simulink model "Gesamtmodell_2015b"  (R2015b)
settings: Solver=ode3  StartTime=0.0  StopTime=inf  FixedStep=dt  RelTol=1e-3
undefined symbols (not defined in the file or in its folder): Com1, dt, K1, K2, K3, Kpsi, Kx, Ky, none, sigbuilder_block, Tpsi, Tx, Ty
libraries: xpcrtudplib x9, xpcobsoletelib x4, simulink x2, xpcseriallib x1, slrtlib x1
(part 1 of 3)
CloseFcn:
  | rtwprivate ssgencode ModelCloseRequest Robotino_Strecke_reall_2009
settings Model: SimulationMode=external  Creator=atlabor  LastModifiedBy=atlabor
settings SolverCC: EnableConcurrentExecution=on
settings DataIOCC: LimitDataPoints=off  SaveFormat=Array  SignalLoggingSaveFormat=ModelDataLogs
settings OptimizationCC: BlockReduction=off  OptimizeBlockIOStorage=off  BufferReuse=off  GlobalBufferReuse=off  ExpressionFolding=off  ExpressionDepthLimit=2147483647  LocalBlockOutputs=off  InitFltsAndDblsToZero=on
settings DebuggingCC: SaveWithParameterizedLinksMsg=none  UnderspecifiedInitializationDetection=Classic  MergeDetectMultiDrivingBlocksExec=none  SolverPrmCheckMsg=warning  FcnCallInpInsideContextMsg=EnableAllAsWarning  StateNameClashWarn=warning
settings HardwareCC: ProdBitPerPointer=32  ProdLargestAtomicFloat=None  ProdWordSize=32  ProdLongLongMode=on  ProdHWDeviceType=Generic->32-bit x86 compatible
settings SFSimCC: SimParseCustomCode=off
settings RTWCC: SystemTargetFile=slrt.tlc  TemplateMakefile=slrt_default_tmf  Description=Simulink Real-Time  RTWCompilerOptimization=on
settings ConfigComp: CovModelRefEnable=Off  CovSFcnEnable=off

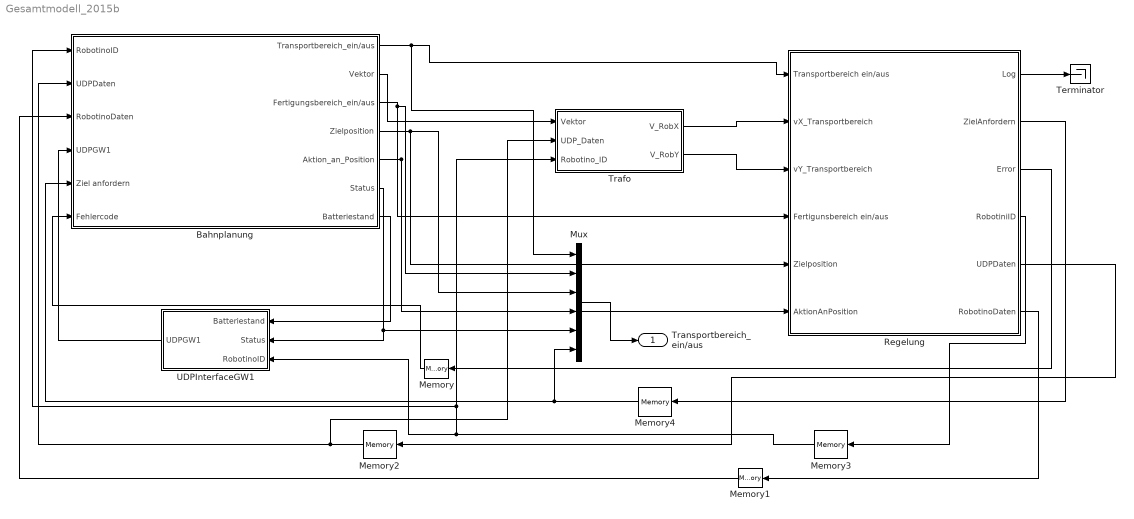
== system Gesamtmodell_2015b ==
  Bahnplanung : Subsystem
  Memory{,1..4} (5 alike) : Memory
  Mux : Mux  Inputs=6
  Regelung : Subsystem
  Terminator : Terminator
  Trafo : MATLAB Function  TreatAsAtomicUnit=on
  UDPInterfaceGW1 : Subsystem
  Transportbereich_ein/aus : Outport
  wires:
  Bahnplanung/1(Transportbereich_ein/aus) -> Mux/1, Regelung/1(Transportbereich ein/aus)
  Bahnplanung/3(Fertigungsbereich_ein/aus) -> Mux/2, Regelung/4(Fertigunsbereich ein/aus)
  Bahnplanung/7(Batteriestand) -> UDPInterfaceGW1/1(Batteriestand)
  Bahnplanung/6(Status) -> UDPInterfaceGW1/2(Status), Mux/5
  UDPInterfaceGW1/1(UDPGW1) -> Bahnplanung/4(UDPGW1)
  Regelung/3(Error) -> Memory/1
  Bahnplanung/4(Zielposition) -> Mux/3, Regelung/5(Zielposition)
  Bahnplanung/5(Aktion_an_Position) -> Mux/4, Regelung/6(AktionAnPosition)
  Regelung/5(UDPDaten) -> Memory2/1
  Regelung/6(RobotinoDaten) -> Memory1/1
  Regelung/1(Log) -> Terminator/1
  Memory/1 -> Bahnplanung/6(Fehlercode)
  Memory1/1 -> Bahnplanung/3(RobotinoDaten)
  Memory3/1 -> UDPInterfaceGW1/3(RobotinoID), Trafo/3(Robotino_ID), Bahnplanung/1(RobotinoID)
  Regelung/2(ZielAnfordern) -> Memory4/1
  Trafo/1(V_RobX) -> Regelung/2(vX_Transportbereich)
  Trafo/2(V_RobY) -> Regelung/3(vY_Transportbereich)
  Bahnplanung/2(Vektor) -> Trafo/1(Vektor)
  Memory2/1 -> Trafo/2(UDP_Daten), Bahnplanung/2(UDPDaten)
  Regelung/4(RobotiniID) -> Memory3/1
  Mux/1 -> Transportbereich_ein/aus/1
  Memory4/1 -> Mux/6, Bahnplanung/5(Ziel anfordern)

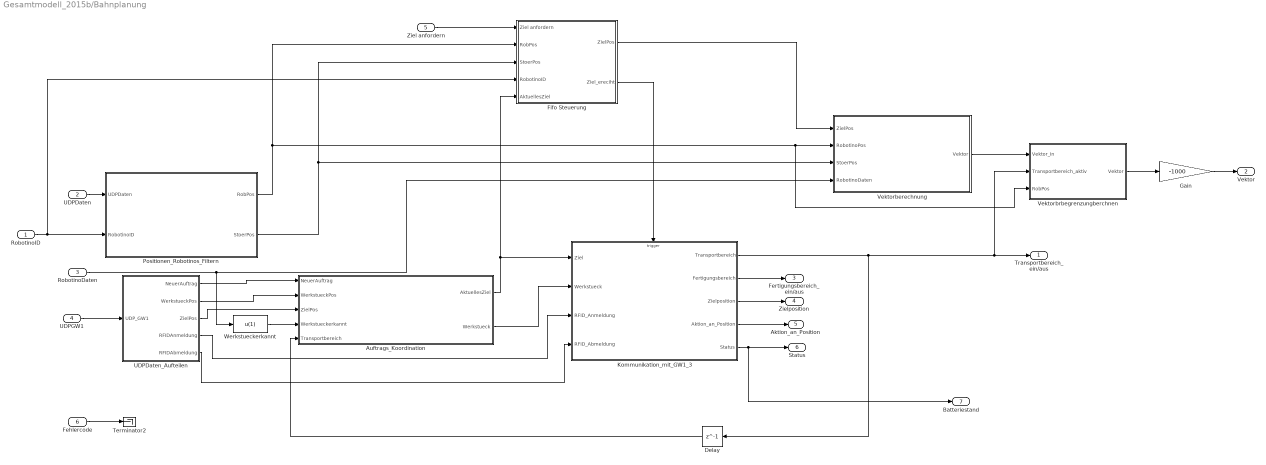
== system Gesamtmodell_2015b/Bahnplanung ==
  RobotinoID : Inport
  UDPDaten : Inport  Port=2  PortDimensions=56
  RobotinoDaten : Inport  Port=3
  UDPGW1 : Inport  Port=4
  Ziel anfordern : Inport  Port=5
  Fehlercode : Inport  Port=6
  Auftrags_Koordination : Stateflow chart  TreatAsAtomicUnit=on
  Delay : Delay  DelayLength=1
  Fifo Steuerung : Subsystem
  Gain : Gain  Gain=-1000
  Kommunikation_mit_GW1_3 : Stateflow chart  TreatAsAtomicUnit=on
  Positionen_Robotinos_Filtern : MATLAB Function  TreatAsAtomicUnit=on
  Terminator2 : Terminator
  UDPDaten_Aufteilen : Subsystem
  Vektorberechnung : Subsystem
  Vektorbrbegrenzungberchnen : MATLAB Function  TreatAsAtomicUnit=on
  Werkstueckerkannt : Fcn  Expr=u(1)
  Transportbereich_ein/aus : Outport
  Vektor : Outport  Port=2  OutDataTypeStr=double  PortDimensions=[1 2]
  Fertigungsbereich_ein/aus : Outport  Port=3
  Zielposition : Outport  Port=4
  Aktion_an_Position : Outport  Port=5
  Status : Outport  Port=6
  Batteriestand : Outport  Port=7
  wires:
  RobotinoID/1 -> Positionen_Robotinos_Filtern/2(RobotinoID), Fifo Steuerung/4(RobotinoID)
  UDPDaten/1 -> Positionen_Robotinos_Filtern/1(UDPDaten)
  Positionen_Robotinos_Filtern/2(StoerPos) -> Fifo Steuerung/3(StoerPos), Vektorberechnung/3(StoerPos)
  RobotinoDaten/1 -> Vektorberechnung/4(RobotinoDaten), Werkstueckerkannt/1
  Kommunikation_mit_GW1_3/3(Zielposition) -> Zielposition/1
  Kommunikation_mit_GW1_3/4(Aktion_an_Position) -> Aktion_an_Position/1
  Kommunikation_mit_GW1_3/2(Fertigungsbereich) -> Fertigungsbereich_ein/aus/1
  Kommunikation_mit_GW1_3/1(Transportbereich) -> Delay/1, Transportbereich_ein/aus/1, Vektorbrbegrenzungberchnen/2(Transportbereich_aktiv)
  UDPGW1/1 -> UDPDaten_Aufteilen/1(UDP_GW1)
  UDPDaten_Aufteilen/4(RFIDAnmeldung) -> Kommunikation_mit_GW1_3/3(RFID_Anmeldung)
  UDPDaten_Aufteilen/5(RFIDAbmeldung) -> Kommunikation_mit_GW1_3/4(RFID_Abmeldung)
  UDPDaten_Aufteilen/2(WerkstueckPos) -> Auftrags_Koordination/2(WerkstueckPos)
  UDPDaten_Aufteilen/3(ZielPos) -> Auftrags_Koordination/3(ZielPos)
  Auftrags_Koordination/1(AktuellesZiel) -> Fifo Steuerung/5(AktuellesZiel), Kommunikation_mit_GW1_3/1(Ziel)
  Fehlercode/1 -> Terminator2/1
  UDPDaten_Aufteilen/1(NeuerAuftrag) -> Auftrags_Koordination/1(NeuerAuftrag)
  Auftrags_Koordination/2(Werkstueck) -> Kommunikation_mit_GW1_3/2(Werkstueck)
  Werkstueckerkannt/1 -> Auftrags_Koordination/4(Werkstueckerkannt)
  Vektorbrbegrenzungberchnen/1(Vektor) -> Gain/1
  Gain/1 -> Vektor/1
  Positionen_Robotinos_Filtern/1(RobPos) -> Vektorbrbegrenzungberchnen/3(RobPos), Vektorberechnung/2(RobotinoPos), Fifo Steuerung/2(RobPos)
  Vektorberechnung/1(Vektor) -> Vektorbrbegrenzungberchnen/1(Vektor_In)
  Ziel anfordern/1 -> Fifo Steuerung/1(Ziel anfordern)
  Fifo Steuerung/1(ZielPos) -> Vektorberechnung/1(ZielPos)
  Fifo Steuerung/2(Ziel_ereciht) -> Kommunikation_mit_GW1_3/Trigger
  Delay/1 -> Auftrags_Koordination/5(Transportbereich)
  Kommunikation_mit_GW1_3/5(Status) -> Batteriestand/1, Status/1

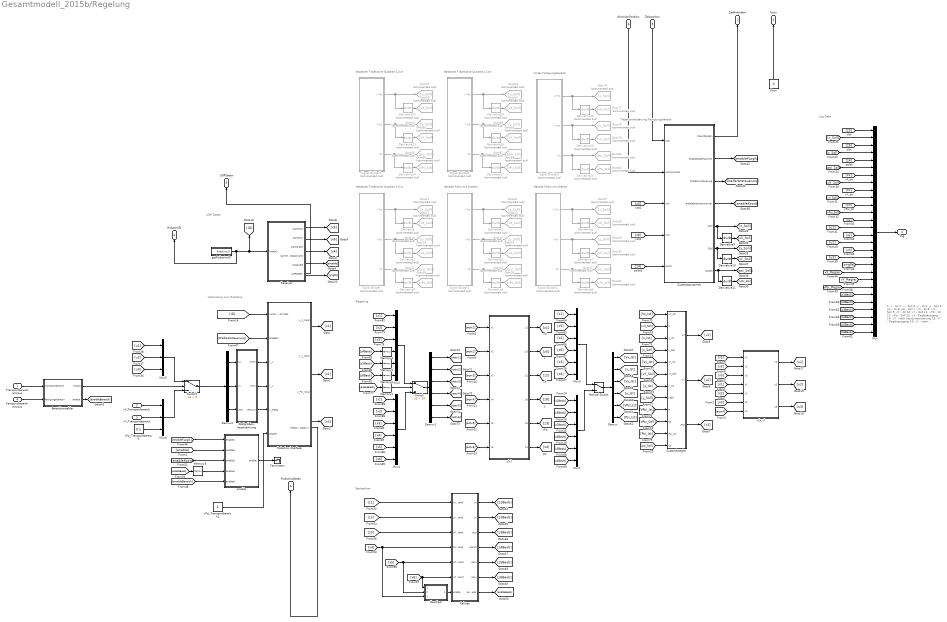
== system Gesamtmodell_2015b/Regelung ==
  note: Trajektorienplanung Fertigungsbereich
  note: Regelung
  note: Verbindung zum Robotino
  note: UDP Daten
  note: Geplante Trajektorie Quadrat 1x1m
  note: Log Data
  note: 1:    x     - Ist
      | 2:    x     - Soll
      | 3:    y     - Ist
      | 4:    y     - Soll
      | 5:   psi   - Ist
      | 6:   psi   - Soll
      | 7:   vX   - Ist
      | 8:   vX   - Soll
      | 9:   vY   - Ist
      | 10: vY   - Soll
      | 11: vPsi - Ist
      | 12: vPsi - Soll
      | 13: vX   - Reglerausgang
      | 14: vX   - nach InputLinearisierung
      | 15: vY   - Reglerausgang
      | 16: vY  - nach InputLinearisierung
      | 17: vPsi - Reglerausgang
      | 18: vPsi - nach InputLinearisierung
      | 19: Kamera Psi
      | 20: vX   - Regler (Geschwindigkeit)
      | 21: vY   - Regler (Geschwindigkeit)
      | 22: vPsi - Regler (Geschwindigkeit)
  note: Gerade Fahrt mit Drehen
  note: Gerade Fahrt mit Drehen
  note: Beobachter
  note: Geplante Trajektorie Quadrat 1x1m
  note: Geplante Trajektorie Quadrat 1x1m
  note: hinter Fertigungsbereich
  Transportbereich ein/aus : Inport
  vX_Transportbereich : Inport  Port=2
  vY_Transportbereich : Inport  Port=3
  Fertigunsbereich ein/aus : Inport  Port=4
  Zielposition : Inport  Port=5
  AktionAnPosition : Inport  Port=6
  Bereichswaehler : MATLAB Function  TreatAsAtomicUnit=on
  Demux : Demux  Outputs=6
  Demux1 : Demux  Outputs=6
  Demux2 : Demux  Outputs=3
  Derivative{,1..8,12..20} (18 alike) : Derivative  Commented=on
  Derivative10 : Derivative
  Derivative11 : Derivative
  Derivative9 : Derivative
  "Error " : Constant  Value=0
  Goto{11,21,27,52,63,76} (6 alike) : Goto  Commented=on  GotoTag=x_Soll
  Goto{12,22,28,53,64,77} (6 alike) : Goto  Commented=on  GotoTag=vX_Soll
  Goto{13,23,29,54,65,78} (6 alike) : Goto  Commented=on  GotoTag=y_Soll
  Goto{14,24,30,55,66,79} (6 alike) : Goto  Commented=on  GotoTag=vY_Soll
  Goto{15,25,31,56,67,80} (6 alike) : Goto  Commented=on  GotoTag=psi_Soll
  Goto{16,26,32,68..69,81} (6 alike) : Goto  Commented=on  GotoTag=vPsi_Soll
  Kalman : MATLAB Function  TreatAsAtomicUnit=on
  Manual Switch : ManualSwitch
  Memory{1..5} (5 alike) : Memory
  Mux : Mux  Inputs=28
  Mux{1..4} (4 alike) : Mux  Inputs=6
  Mux5 : Mux  Inputs=3
  Mux6 : Mux  Inputs=3
  NewCam : MATLAB Function  TreatAsAtomicUnit=on
  Receiver : Subsystem
  Robotino interface : Subsystem
  Signal Builder : Subsystem  Tag=STV Subsys  Commented=on  LoadFcn=sigbuilder_block('load');  StartFcn=sigbuilder_block('start');  StopFcn=sigbuilder_block('stop');  ClipboardFcn=sigbuilder_block('clipboard');  mask(Sigbuilder block){}
      mask help: Simulink:masks:SigbuilderBlock_MD
      mask init:
      | if ~strcmp(get_param(bdroot(gcbh),'SimulationStatus'),'stopped') tuvar = sigbuilder_block('maskInit'); end
      settings: CopyFcn=sigbuilder_block('copy');  DeleteFcn=sigbuilder_block('delete');  ModelCloseFcn=sigbuilder_block('modelClose');  PreSaveFcn=sigbuilder_block('preSave');  PauseFcn=sigbuilder_block('pause');  ContinueFcn=sigbuilder_block('continue');  NameChangeFcn=sigbuilder_block('namechange');  OpenFcn=sigbuilder_block('open',[6 30 1248 660 ]);  CloseFcn=sigbuilder_block('close');
      mask Display: plot(0, 0, 100, 100,[2, 2, 32, 32, 2], [68, 8, 8, 68, 68],[32, 2], [38, 38], [32, 19, 2],[53, 60, 44], [32, 17, 17, 2],[16, 16, 31, 31]);txt = getActiveGroup(gcbh);text(2, 100, txt,'verticalAlignment', 'top');
  Signal Builder1 : Subsystem  Tag=STV Subsys  Commented=on  LoadFcn=sigbuilder_block('load');  StartFcn=sigbuilder_block('start');  StopFcn=sigbuilder_block('stop');  ClipboardFcn=sigbuilder_block('clipboard');  mask(Sigbuilder block){}
      mask help: Simulink:masks:SigbuilderBlock_MD
      mask init:
      | if ~strcmp(get_param(bdroot(gcbh),'SimulationStatus'),'stopped') tuvar = sigbuilder_block('maskInit'); end
      settings: CopyFcn=sigbuilder_block('copy');  DeleteFcn=sigbuilder_block('delete');  ModelCloseFcn=sigbuilder_block('modelClose');  PreSaveFcn=sigbuilder_block('preSave');  PauseFcn=sigbuilder_block('pause');  ContinueFcn=sigbuilder_block('continue');  NameChangeFcn=sigbuilder_block('namechange');  OpenFcn=sigbuilder_block('open',[6 30 1248 660 ]);  CloseFcn=sigbuilder_block('close');
      mask Display: plot(0, 0, 100, 100,[2, 2, 32, 32, 2], [68, 8, 8, 68, 68],[32, 2], [38, 38], [32, 19, 2],[53, 60, 44], [32, 17, 17, 2],[16, 16, 31, 31]);txt = getActiveGroup(gcbh);text(2, 100, txt,'verticalAlignment', 'top');
  Signal Builder2 : Subsystem  Tag=STV Subsys  Commented=on  LoadFcn=sigbuilder_block('load');  StartFcn=sigbuilder_block('start');  StopFcn=sigbuilder_block('stop');  ClipboardFcn=sigbuilder_block('clipboard');  mask(Sigbuilder block){}
      mask help: Simulink:masks:SigbuilderBlock_MD
      mask init:
      | if ~strcmp(get_param(bdroot(gcbh),'SimulationStatus'),'stopped') tuvar = sigbuilder_block('maskInit'); end
      settings: CopyFcn=sigbuilder_block('copy');  DeleteFcn=sigbuilder_block('delete');  ModelCloseFcn=sigbuilder_block('modelClose');  PreSaveFcn=sigbuilder_block('preSave');  PauseFcn=sigbuilder_block('pause');  ContinueFcn=sigbuilder_block('continue');  NameChangeFcn=sigbuilder_block('namechange');  OpenFcn=sigbuilder_block('open',[6 30 1248 660 ]);  CloseFcn=sigbuilder_block('close');
      mask Display: plot(0, 0, 100, 100,[2, 2, 32, 32, 2], [68, 8, 8, 68, 68],[32, 2], [38, 38], [32, 19, 2],[53, 60, 44], [32, 17, 17, 2],[16, 16, 31, 31]);txt = getActiveGroup(gcbh);text(2, 100, txt,'verticalAlignment', 'top');
  Signal Builder3 : Subsystem  Tag=STV Subsys  Commented=on  LoadFcn=sigbuilder_block('load');  StartFcn=sigbuilder_block('start');  StopFcn=sigbuilder_block('stop');  ClipboardFcn=sigbuilder_block('clipboard');  mask(Sigbuilder block){}
      mask help: Simulink:masks:SigbuilderBlock_MD
      mask init:
      | if ~strcmp(get_param(bdroot(gcbh),'SimulationStatus'),'stopped') tuvar = sigbuilder_block('maskInit'); end
      settings: CopyFcn=sigbuilder_block('copy');  DeleteFcn=sigbuilder_block('delete');  ModelCloseFcn=sigbuilder_block('modelClose');  PreSaveFcn=sigbuilder_block('preSave');  PauseFcn=sigbuilder_block('pause');  ContinueFcn=sigbuilder_block('continue');  NameChangeFcn=sigbuilder_block('namechange');  OpenFcn=sigbuilder_block('open',[6 30 1248 660 ]);  CloseFcn=sigbuilder_block('close');
      mask Display: plot(0, 0, 100, 100,[2, 2, 32, 32, 2], [68, 8, 8, 68, 68],[32, 2], [38, 38], [32, 19, 2],[53, 60, 44], [32, 17, 17, 2],[16, 16, 31, 31]);txt = getActiveGroup(gcbh);text(2, 100, txt,'verticalAlignment', 'top');
  Signal Builder4 : Subsystem  Tag=STV Subsys  Commented=on  LoadFcn=sigbuilder_block('load');  StartFcn=sigbuilder_block('start');  StopFcn=sigbuilder_block('stop');  ClipboardFcn=sigbuilder_block('clipboard');  mask(Sigbuilder block){}
      mask help: Simulink:masks:SigbuilderBlock_MD
      mask init:
      | if ~strcmp(get_param(bdroot(gcbh),'SimulationStatus'),'stopped') tuvar = sigbuilder_block('maskInit'); end
      settings: CopyFcn=sigbuilder_block('copy');  DeleteFcn=sigbuilder_block('delete');  ModelCloseFcn=sigbuilder_block('modelClose');  PreSaveFcn=sigbuilder_block('preSave');  PauseFcn=sigbuilder_block('pause');  ContinueFcn=sigbuilder_block('continue');  NameChangeFcn=sigbuilder_block('namechange');  OpenFcn=sigbuilder_block('open',[6 30 1248 660 ]);  CloseFcn=sigbuilder_block('close');
      mask Display: plot(0, 0, 100, 100,[2, 2, 32, 32, 2], [68, 8, 8, 68, 68],[32, 2], [38, 38], [32, 19, 2],[53, 60, 44], [32, 17, 17, 2],[16, 16, 31, 31]);txt = getActiveGroup(gcbh);text(2, 100, txt,'verticalAlignment', 'top');
  Signal Builder5 : Subsystem  Tag=STV Subsys  Commented=on  LoadFcn=sigbuilder_block('load');  StartFcn=sigbuilder_block('start');  StopFcn=sigbuilder_block('stop');  ClipboardFcn=sigbuilder_block('clipboard');  mask(Sigbuilder block){}
      mask help: Simulink:masks:SigbuilderBlock_MD
      mask init:
      | if ~strcmp(get_param(bdroot(gcbh),'SimulationStatus'),'stopped') tuvar = sigbuilder_block('maskInit'); end
      settings: CopyFcn=sigbuilder_block('copy');  DeleteFcn=sigbuilder_block('delete');  ModelCloseFcn=sigbuilder_block('modelClose');  PreSaveFcn=sigbuilder_block('preSave');  PauseFcn=sigbuilder_block('pause');  ContinueFcn=sigbuilder_block('continue');  NameChangeFcn=sigbuilder_block('namechange');  OpenFcn=sigbuilder_block('open',[6 30 1248 660 ]);  CloseFcn=sigbuilder_block('close');
      mask Display: plot(0, 0, 100, 100,[2, 2, 32, 32, 2], [68, 8, 8, 68, 68],[32, 2], [38, 38], [32, 19, 2],[53, 60, 44], [32, 17, 17, 2],[16, 16, 31, 31]);txt = getActiveGroup(gcbh);text(2, 100, txt,'verticalAlignment', 'top');
  "Stellgrößen- beschränkung " : Subsystem
  Switch : Switch  Criteria=u2 > Threshold  Threshold=10
  Switch1 : Switch  Criteria=u2 > Threshold
  Terminator : Terminator
  Zustandsautomat : Subsystem
  Zustandsregler : Subsystem
  "enable " : MATLAB Function  TreatAsAtomicUnit=on
  getRobotinoID : Subsystem
  "u(x,v) " : MATLAB Function  TreatAsAtomicUnit=on
  vPsi_Transportbereich : Constant  Value=0.1
  vPsi_Transportbereich1 : Constant
  z(x) : MATLAB Function  TreatAsAtomicUnit=on
  Log : Outport
  ZielAnfordern : Outport  Port=2
  Error : Outport  Port=3
  RobotiniID : Outport  Port=4
  UDPDaten : Outport  Port=5
  RobotinoDaten : Outport  Port=6
  wires:
  Fertigunsbereich ein/aus/1 -> Bereichswaehler/2(fertigungsbereich)
  Bereichswaehler/2(enable) -> [enableBereich]
  "Error "/1 -> Error/1
  Mux5/1 -> Switch1/1
  [u1] -> Mux5/1
  [GreiferAnsteuerung] -> Robotino interface/2(Grabber)
  Mux/1 -> Log/1
  [enableBereich] -> "enable "/5(enable5)
  Derivative4/1 -> Goto16/1
  Signal Builder/1(X Pos) -> Derivative/1, Goto11/1
  [u2] -> Mux5/2
  [u3] -> Mux5/3
  vPsi_Transportbereich/1 -> Mux6/3
  Zustandsautomat/1(ZielAnfordern) -> ZielAnfordern/1
  Transportbereich ein/aus/1 -> Bereichswaehler/1(transportbereich)
  Mux6/1 -> Switch1/3
  Bereichswaehler/1(modus) -> Switch1/2
  [x3] -> Mux2/3
  [x1] -> "u(x,v) "/4(x1)
  [x3] -> "u(x,v) "/6(x3)
  [z1] -> Mux/7
  [u2] -> Mux/16
  Receiver/5("origAngle ") -> [origPsi]
  Demux2/2 -> "Stellgrößen- beschränkung "/2(vY)
  Demux2/3 -> "Stellgrößen- beschränkung "/3(vPsi)
  Mux1/1 -> Manual Switch/2
  Mux3/1 -> Manual Switch/1
  [v3] -> "u(x,v) "/3(v3)
  Signal Builder5/3(Psi) -> Goto80/1, Derivative20/1
  [z3] -> Kalman/3(vPsiZustand)
  [u3] -> Mux/18
  [z4] -> Mux3/6
  [z1Beob] -> Mux1/1
  [z5Beob] -> Mux1/2
  [z6Beob] -> Mux1/4
  [u1] -> Mux/14
  Signal Builder1/1(X Pos) -> Derivative1/1, Goto21/1
  [origPsi] -> Mux/19
  [z5] -> Mux/1
  "Stellgrößen- beschränkung "/1(vXlim) -> Robotino interface/3(v_x)
  Derivative11/1 -> [vPsi_Soll]
  Derivative10/1 -> [vY_Soll]
  Signal Builder2/3(Psi) -> Derivative8/1, Goto31/1
  Derivative7/1 -> Goto30/1
  Signal Builder3/3(Psi) -> Goto56/1, Derivative14/1
  Signal Builder1/2(Y Pos) -> Derivative2/1, Goto23/1
  [z6] -> Zustandsautomat/4(yIst)
  Zustandsautomat/2(enableStateMachine) -> [enableFLogik]
  [v3] -> Mux/17
  Receiver/4(CameraSignalValid) -> [enable]
  [psi_Soll] -> Zustandsregler/12("psi_Soll ")
  [z6] -> Mux/3
  Receiver/3("CameraPsi ") -> [x4]
  [vPsi_Soll] -> Mux/12
  z(x)/6(z4) -> [z4]
  vX_Transportbereich/1 -> Mux6/1
  [z2Beob] -> Mux/24
  [z6Beob] -> Mux/28
  [z2] -> Mux3/3
  [z5] -> Mux3/2
  [z4Beob] -> Mux1/6
  [vY_Soll] -> Mux/10
  [vX_Soll] -> Mux/8
  Signal Builder4/3(Psi) -> Goto67/1, Derivative17/1
  Derivative9/1 -> [vX_Soll]
  Memory5/1 -> "enable "/4(enable4)
  Robotino interface/3("v_Psi_lokal ") -> [x3]
  [x2] -> "u(x,v) "/5(x2)
  Robotino interface/2("v_Y_lokal ") -> [x2]
  z(x)/2(z5) -> [z5]
  [z3] -> Mux/11
  [z2] -> Mux/9
  [x5] -> Kalman/5(xZustand), NewCam/2(xZustand)
  Zustandsregler/1(vX) -> [v1]
  Zustandsregler/2(vY) -> [v2]
  Kalman/2(vy) -> [z2Beob]
  [z3Beob] -> Mux/25
  [Psi_Ist] -> Zustandsregler/11(Psi_ist)
  [z1] -> Kalman/1(vxZustand)
  [VPsi_Ist] -> Zustandsregler/9(vPsi_ist)
  Zustandsautomat/3(GreiferAnsteuerung) -> [GreiferAnsteuerung]
  vY_Transportbereich/1 -> Mux6/2
  [x2] -> Mux2/2
  Mux4/1 -> Switch/3
  Demux1/2 -> [actx2]
  Demux1/1 -> [actx1]
  Kalman/4(pospsi) -> [z4Beob]
  [z3Beob] -> Mux1/5
  NewCam/1(enable) -> Kalman/7(enable)
  [ID] -> Robotino interface/1(number of robot)
  Zustandsregler/3("vPsi ") -> [v3]
  Manual Switch/1 -> Demux/1
  Memory4/1 -> Mux2/4
  [enableBeob] -> Memory1/1
  [x6] -> NewCam/1(yZustand), Kalman/6(yZustand)
  Signal Builder3/2(Y Pos) -> Goto54/1, Derivative13/1
  [vY_Soll] -> Zustandsregler/6("vY_Soll ")
  Derivative/1 -> Goto12/1
  [x_Soll] -> Zustandsregler/4(x_Soll)
  Demux1/3 -> [actx3]
  [vY_Regler] -> Mux/21
  Zustandsautomat/6(YSoll) -> [y_Soll], Derivative10/1
  [vX_Soll] -> Zustandsregler/2("vX_Soll ")
  "Stellgrößen- beschränkung "/3(vPsiLim) -> Robotino interface/5(v_theta)
  z(x)/4(z6) -> [z6]
  z(x)/5(z3) -> [z3]
  Zustandsautomat/7(psiSoll) -> [psi_Soll], Derivative11/1
  [enableFLogik] -> "enable "/1(enable1)
  [z5] -> Zustandsautomat/3(xIst)
  AktionAnPosition/1 -> Zustandsautomat/2(AktionAnZiel)
  [z4Beob] -> Mux/26
  [z5Beob] -> Mux/27
  [z2] -> Kalman/2(vyZustand)
  Signal Builder4/1(X Pos) -> Goto63/1, Derivative15/1
  Zustandsautomat/5(xSoll) -> Derivative9/1, [x_Soll]
  Mux2/1 -> Switch/1
  Switch/1 -> Demux1/1
  [actx2] -> z(x)/2(x2)
  [actx3] -> z(x)/3(x3)
  [actx5] -> z(x)/5(x5)
  [actx1] -> z(x)/1(x1)
  Zielposition/1 -> Zustandsautomat/1("Ziel ")
  [z4] -> Zustandsautomat/5(psiIst)
  [z3] -> Mux3/5
  Demux/1 -> [Vx_Ist]
  Signal Builder4/2(Y Pos) -> Goto65/1, Derivative16/1
  [actx6] -> z(x)/6(x6)
  Receiver/1(CameraX) -> [x5]
  Receiver/2(CameraY) -> [x6]
  [vPsi_Soll] -> Zustandsregler/10(vPsi_Soll)
  [x_Soll] -> Mux/2
  [x4] -> Mux4/4
  [x5] -> Mux4/5
  Signal Builder3/1(X Pos) -> Goto52/1, Derivative12/1
  [y_Soll] -> Zustandsregler/8(ySoll)
  Demux1/5 -> [actx5]
  Demux1/4 -> [actx4]
  [z6Beob] -> Memory2/1
  Demux1/6 -> [actx6]
  Zustandsautomat/4(enableStationsnummer) -> [enableKoord]
  [enableKoord] -> "enable "/3(enable3)
  Robotino interface/1(v_X_lokal) -> [x1]
  "Stellgrößen- beschränkung "/2(vYlim) -> Robotino interface/4(v_y)
  z(x)/1(z1) -> [z1]
  Derivative18/1 -> Goto77/1
  Derivative19/1 -> Goto79/1
  Derivative20/1 -> Goto81/1
  Memory3/1 -> Mux2/5
  [z4Beob] -> Memory4/1
  [enableBeob] -> Memory5/1
  Derivative12/1 -> Goto53/1
  Derivative14/1 -> Goto69/1
  Derivative8/1 -> Goto32/1
  [vPsi_Regler] -> Mux/22
  Demux/2 -> [x_Ist]
  [Vx_Ist] -> Zustandsregler/1(vX_Ist)
  Signal Builder/2(Y Pos) -> Derivative3/1, Goto13/1
  Kalman/6(posy) -> [z6Beob]
  Kalman/1(vx) -> [z1Beob]
  Kalman/5(posx) -> [z5Beob]
  Memory1/1 -> Switch/2
  Signal Builder5/1(X Pos) -> Goto76/1, Derivative18/1
  [psi_Soll] -> Mux/6
  z(x)/3(z2) -> [z2]
  [v2] -> "u(x,v) "/2(v2)
  [v1] -> "u(x,v) "/1(v1)
  [z1] -> Mux3/1
  [z6] -> Mux3/4
  "u(x,v) "/2(u2) -> [u2]
  "u(x,v) "/3(u3) -> [u3]
  "u(x,v) "/1(u1) -> [u1]
  [v1] -> Mux/13
  [v2] -> Mux/15
  Derivative15/1 -> Goto64/1
  Derivative17/1 -> Goto68/1
  Derivative16/1 -> Goto66/1
  Derivative13/1 -> Goto55/1
  [z2Beob] -> Mux1/3
  [z1Beob] -> Mux/23
  Kalman/3(vpsi) -> [z3Beob]
  Derivative2/1 -> Goto24/1
  Signal Builder/3(Psi) -> Derivative4/1, Goto15/1
  Derivative3/1 -> Goto14/1
  getRobotinoID/1(Robotino.ID) -> [ID], Receiver/1("RoboID "), RobotiniID/1
  [actx4] -> z(x)/4(x4)
  Kalman/7(enableBeob) -> [enableBeob]
  [x1] -> Mux4/1
  [x3] -> Mux4/3
  [x2] -> Mux4/2
  Derivative6/1 -> Goto28/1
  Signal Builder2/2(Y Pos) -> Derivative7/1, Goto29/1
  Signal Builder5/2(Y Pos) -> Goto78/1, Derivative19/1
  [x6] -> Mux4/6
  [x1] -> Mux2/1
  [x4] -> Kalman/4(PsiZustand), NewCam/3(psiZustand)
  Derivative5/1 -> Goto26/1
  Demux2/1 -> "Stellgrößen- beschränkung "/1(vX)
  [actx4] -> "u(x,v) "/7(x4)
  Demux/4 -> [y_Ist]
  Demux/3 -> [Vy_Ist]
  Memory2/1 -> Mux2/6
  [z5Beob] -> Memory3/1
  Signal Builder2/1(X Pos) -> Derivative6/1, Goto27/1
  Signal Builder1/3(Psi) -> Derivative5/1, Goto25/1
  Demux/5 -> [VPsi_Ist]
  Demux/6 -> [Psi_Ist]
  [x_Ist] -> Zustandsregler/3(x_Ist)
  Derivative1/1 -> Goto22/1
  [y_Soll] -> Mux/4
  [z4] -> Mux/5
  [enable] -> "enable "/2(enable2)
  [vX_Regler] -> Mux/20
  [Vy_Ist] -> Zustandsregler/5(vY_Ist)
  [y_Ist] -> Zustandsregler/7(y_Ist)
  Receiver/6(UDPDaten) -> UDPDaten/1
  Robotino interface/4(RobotinoDaten 1) -> RobotinoDaten/1
  vPsi_Transportbereich1/1 -> Robotino interface/6(enable)
  "enable "/1(enable) -> Terminator/1
  Switch1/1 -> Demux2/1

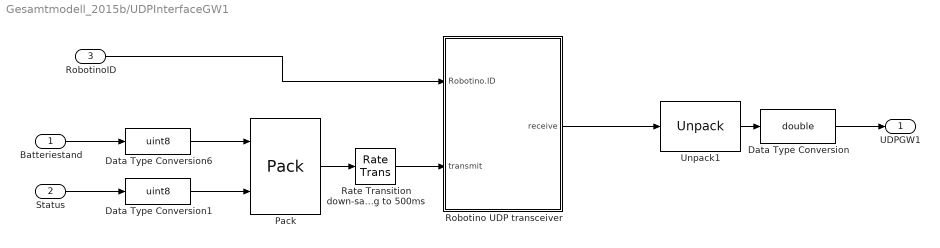
== system Gesamtmodell_2015b/UDPInterfaceGW1 ==
  Batteriestand : Inport
  Status : Inport  Port=2
  RobotinoID : Inport  Port=3
  Data Type Conversion : DataTypeConversion  OutDataTypeStr=double
  Data Type Conversion1 : DataTypeConversion  OutDataTypeStr=uint8
  Data Type Conversion6 : DataTypeConversion  OutDataTypeStr=uint8
  Pack : xpcobsoletelib/Utilities/Pack   datatypes={'uint8','uint8'}  byteAlign=1
  Rate Transition down-sampling to 500ms : RateTransition  OutPortSampleTime=0.5
  Robotino UDP transceiver : Subsystem
  Unpack1 : xpcobsoletelib/Utilities/Unpack   dimensions={[8]}  datatypes={'int8'}  byteAlign=1
  UDPGW1 : Outport
  wires:
  Pack/1 -> Rate Transition down-sampling to 500ms/1
  Data Type Conversion1/1 -> Pack/2
  Data Type Conversion6/1 -> Pack/1
  Batteriestand/1 -> Data Type Conversion6/1
  Status/1 -> Data Type Conversion1/1
  Robotino UDP transceiver/1(receive) -> Unpack1/1
  Rate Transition down-sampling to 500ms/1 -> Robotino UDP transceiver/2(transmit)
  RobotinoID/1 -> Robotino UDP transceiver/1(Robotino.ID)
  Unpack1/1 -> Data Type Conversion/1
  Data Type Conversion/1 -> UDPGW1/1

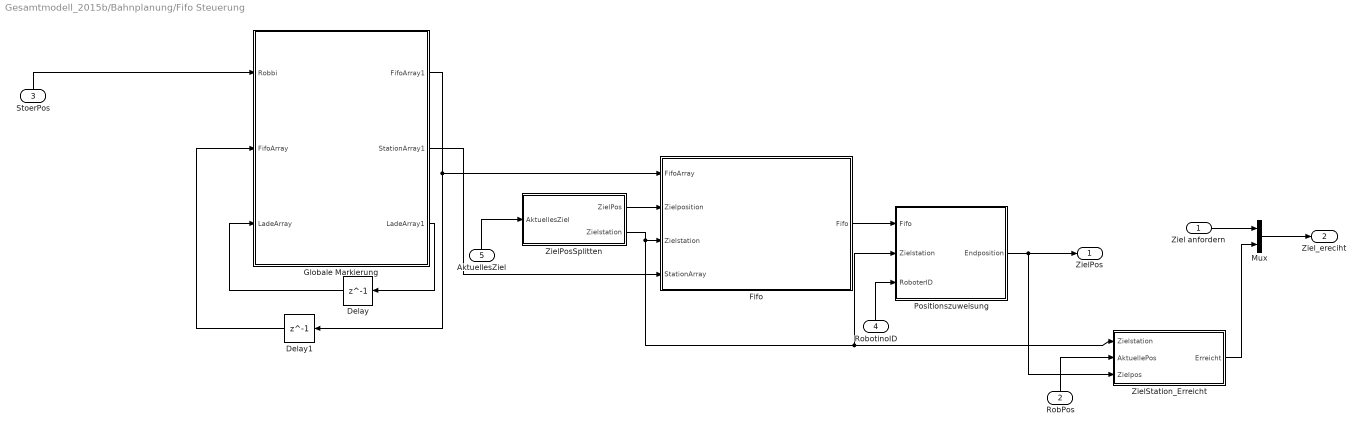
== system Gesamtmodell_2015b/Bahnplanung/Fifo Steuerung ==
  Ziel anfordern : Inport
  RobPos : Inport  Port=2
  StoerPos : Inport  Port=3
  RobotinoID : Inport  Port=4
  AktuellesZiel : Inport  Port=5
  Delay : Delay  DelayLength=1
  Delay1 : Delay  DelayLength=1
  Fifo : Stateflow chart  TreatAsAtomicUnit=on
  Globale Markierung : MATLAB Function  TreatAsAtomicUnit=on
  Mux : Mux  Inputs=2
  Positionszuweisung : MATLAB Function  TreatAsAtomicUnit=on
  ZielPosSplitten : MATLAB Function  TreatAsAtomicUnit=on
  ZielStation_Erreicht : MATLAB Function  TreatAsAtomicUnit=on
  ZielPos : Outport
  Ziel_ereciht : Outport  Port=2
  wires:
  RobotinoID/1 -> Positionszuweisung/3(RoboterID)
  RobPos/1 -> ZielStation_Erreicht/2(AktuellePos)
  StoerPos/1 -> Globale Markierung/1(Robbi)
  AktuellesZiel/1 -> ZielPosSplitten/1(AktuellesZiel)
  Positionszuweisung/1(Endposition) -> ZielStation_Erreicht/3(Zielpos), ZielPos/1
  Globale Markierung/2(StationArray1) -> Fifo/4(StationArray)
  ZielPosSplitten/1(ZielPos) -> Fifo/2(Zielposition)
  ZielPosSplitten/2(Zielstation) -> Positionszuweisung/2(Zielstation), ZielStation_Erreicht/1(Zielstation), Fifo/3(Zielstation)
  Globale Markierung/1(FifoArray1) -> Delay1/1, Fifo/1(FifoArray)
  Delay1/1 -> Globale Markierung/2(FifoArray)
  Fifo/1(Fifo) -> Positionszuweisung/1(Fifo)
  Globale Markierung/3(LadeArray1) -> Delay/1
  Delay/1 -> Globale Markierung/3(LadeArray)
  Mux/1 -> Ziel_ereciht/1
  Ziel anfordern/1 -> Mux/1
  ZielStation_Erreicht/1(Erreicht) -> Mux/2

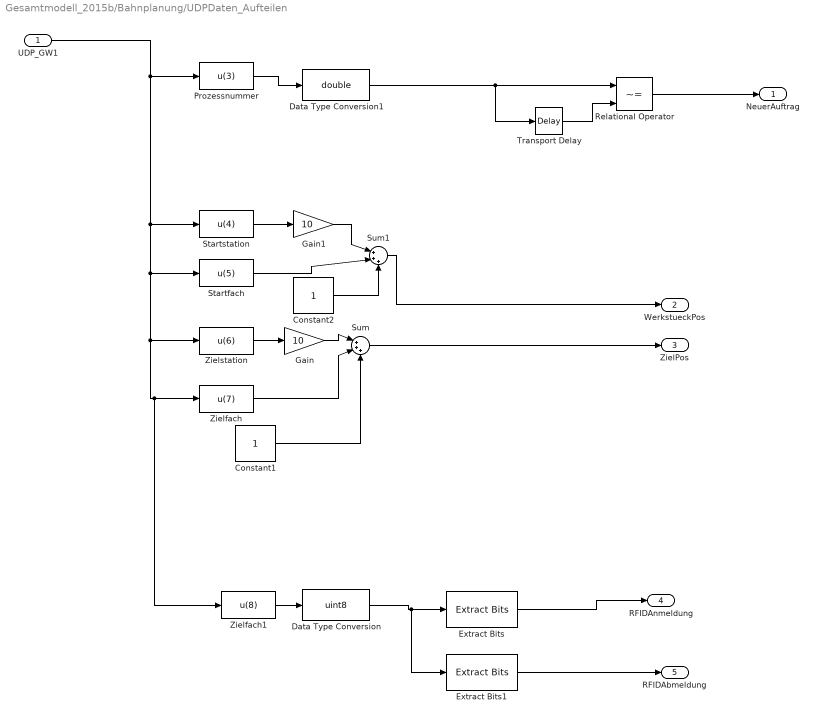
== system Gesamtmodell_2015b/Bahnplanung/UDPDaten_Aufteilen ==
  UDP_GW1 : Inport
  Constant1 : Constant
  Constant2 : Constant
  Data Type Conversion : DataTypeConversion  OutDataTypeStr=uint8
  Data Type Conversion1 : DataTypeConversion  OutDataTypeStr=double
  Extract Bits : simulink/Logic and Bit Operations/Extract Bits  bitsToExtract=Range of bits  numBits=8  bitIdxRange=[0]  outScalingMode=Treat bit field as an integer
  Extract Bits1 : simulink/Logic and Bit Operations/Extract Bits  bitsToExtract=Range of bits  numBits=8  bitIdxRange=[1]  outScalingMode=Treat bit field as an integer
  Gain : Gain  Gain=10
  Gain1 : Gain  Gain=10
  Prozessnummer : Fcn  Expr=u(3)
  Relational Operator : RelationalOperator  Operator=~=  OutDataTypeStr=boolean
  Startfach : Fcn  Expr=u(5)
  Startstation : Fcn  Expr=u(4)
  Sum : Sum  Inputs=|+++
  Sum1 : Sum  Inputs=|+++
  Transport Delay : TransportDelay
  Zielfach : Fcn  Expr=u(7)
  Zielfach1 : Fcn  Expr=u(8)
  Zielstation : Fcn  Expr=u(6)
  NeuerAuftrag : Outport
  WerkstueckPos : Outport  Port=2
  ZielPos : Outport  Port=3
  RFIDAnmeldung : Outport  Port=4
  RFIDAbmeldung : Outport  Port=5
  wires:
  Zielfach/1 -> Sum/2
  Gain/1 -> Sum/1
  Zielstation/1 -> Gain/1
  UDP_GW1/1 -> Prozessnummer/1, Zielfach1/1, Zielfach/1, Zielstation/1, Startfach/1, Startstation/1
  Sum1/1 -> WerkstueckPos/1
  Startfach/1 -> Sum1/2
  Gain1/1 -> Sum1/1
  Constant2/1 -> Sum1/3
  Startstation/1 -> Gain1/1
  Constant1/1 -> Sum/3
  Sum/1 -> ZielPos/1
  Relational Operator/1 -> NeuerAuftrag/1
  Zielfach1/1 -> Data Type Conversion/1
  Data Type Conversion/1 -> Extract Bits1/1, Extract Bits/1
  Data Type Conversion1/1 -> Transport Delay/1, Relational Operator/1
  Transport Delay/1 -> Relational Operator/2
  Extract Bits1/1 -> RFIDAbmeldung/1
  Extract Bits/1 -> RFIDAnmeldung/1
  Prozessnummer/1 -> Data Type Conversion1/1

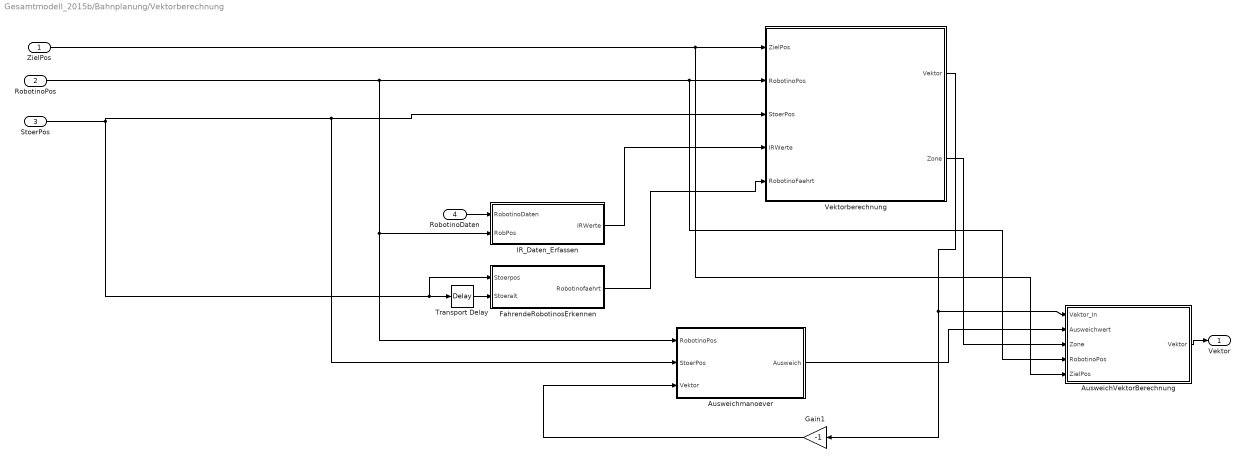
== system Gesamtmodell_2015b/Bahnplanung/Vektorberechnung ==
  ZielPos : Inport
  RobotinoPos : Inport  Port=2
  StoerPos : Inport  Port=3
  RobotinoDaten : Inport  Port=4
  AusweichVektorBerechnung : MATLAB Function  TreatAsAtomicUnit=on
  Ausweichmanoever : MATLAB Function  TreatAsAtomicUnit=on
  FahrendeRobotinosErkennen : MATLAB Function  TreatAsAtomicUnit=on
  Gain1 : Gain  Gain=-1
  IR_Daten_Erfassen : MATLAB Function  TreatAsAtomicUnit=on
  Transport Delay : TransportDelay
  Vektorberechnung : MATLAB Function  TreatAsAtomicUnit=on
  Vektor : Outport
  wires:
  RobotinoPos/1 -> AusweichVektorBerechnung/4(RobotinoPos), Vektorberechnung/2(RobotinoPos), IR_Daten_Erfassen/2(RobPos), Ausweichmanoever/1(RobotinoPos)
  RobotinoDaten/1 -> IR_Daten_Erfassen/1(RobotinoDaten)
  StoerPos/1 -> FahrendeRobotinosErkennen/1(Stoerpos), Transport Delay/1, Vektorberechnung/3(StoerPos), Ausweichmanoever/2(StoerPos)
  ZielPos/1 -> AusweichVektorBerechnung/5(ZielPos), Vektorberechnung/1(ZielPos)
  Ausweichmanoever/1(Ausweich) -> AusweichVektorBerechnung/2(Ausweichwert)
  Vektorberechnung/1(Vektor) -> Gain1/1, AusweichVektorBerechnung/1(Vektor_In)
  Gain1/1 -> Ausweichmanoever/3(Vektor)
  IR_Daten_Erfassen/1(IRWerte) -> Vektorberechnung/4(IRWerte)
  AusweichVektorBerechnung/1(Vektor) -> Vektor/1
  Vektorberechnung/2(Zone) -> AusweichVektorBerechnung/3(Zone)
  FahrendeRobotinosErkennen/1(Robotinofaehrt) -> Vektorberechnung/5(RobotinoFaehrt)
  Transport Delay/1 -> FahrendeRobotinosErkennen/2(Stoeralt)

== system Gesamtmodell_2015b/Regelung/Receiver ==
  "RoboID " : Inport
  Terminator4 : Terminator
  UDP interface : Subsystem
  autoRobID : MATLAB Function  TreatAsAtomicUnit=on
  x4(psi) : MATLAB Function  TreatAsAtomicUnit=on
  CameraX : Outport
  CameraY : Outport  Port=2
  "CameraPsi " : Outport  Port=3
  CameraSignalValid : Outport  Port=4
  "origAngle " : Outport  Port=5
  UDPDaten : Outport  Port=6
  wires:
  autoRobID/1(pX) -> CameraX/1
  autoRobID/4(enable) -> CameraSignalValid/1
  x4(psi)/1(x4) -> "CameraPsi "/1
  autoRobID/2(pY) -> CameraY/1
  autoRobID/3(psi) -> "origAngle "/1, x4(psi)/1(psi)
  UDP interface/2(UDP data) -> UDPDaten/1, autoRobID/1(udpIn)  "56 elements"
  UDP interface/1(enable) -> Terminator4/1  "1 -> permission granted;        0 -> not granted"
  "RoboID "/1 -> autoRobID/2(robID), UDP interface/1(number of robot)

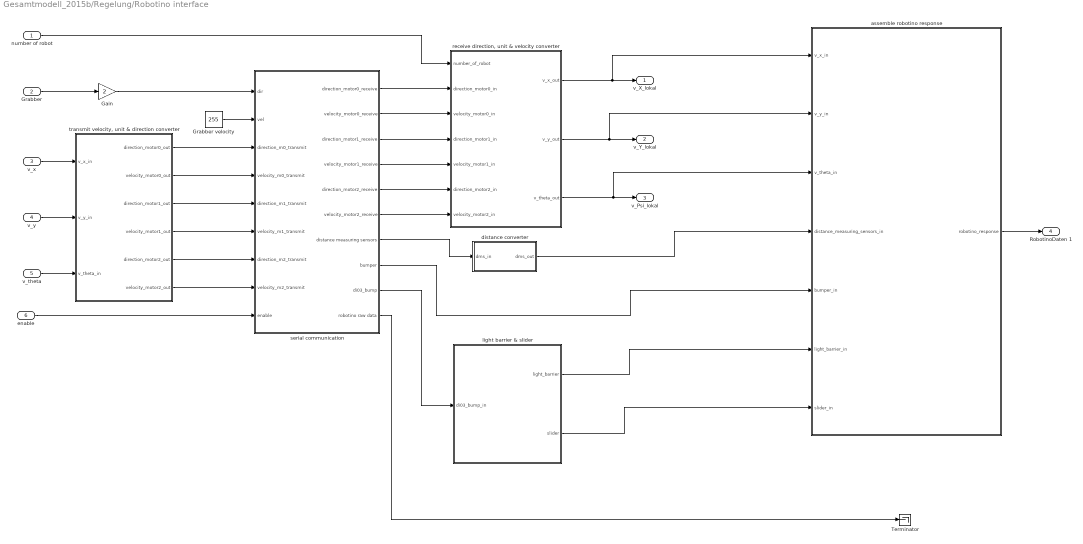
== system Gesamtmodell_2015b/Regelung/Robotino interface ==
  number of robot : Inport
  Grabber : Inport  Port=2
  v_x : Inport  Port=3
  v_y : Inport  Port=4
  v_theta : Inport  Port=5
  enable : Inport  Port=6
  Gain : Gain  Gain=2
  Grabber velocity : Constant  Value=255
  Terminator : Terminator
  assemble robotino response : MATLAB Function  TreatAsAtomicUnit=on
  distance converter : MATLAB Function  TreatAsAtomicUnit=on
  light barrier & slider : MATLAB Function  TreatAsAtomicUnit=on
  "receive direction, unit & velocity converter" : MATLAB Function  TreatAsAtomicUnit=on
  serial communication : Subsystem
  "transmit velocity, unit & direction converter" : MATLAB Function  TreatAsAtomicUnit=on
  v_X_lokal : Outport
  "v_Y_lokal " : Outport  Port=2
  "v_Psi_lokal " : Outport  Port=3
  RobotinoDaten 1 : Outport  Port=4
  wires:
  "transmit velocity, unit & direction converter"/1(direction_motor0_out) -> serial communication/3(direction_m0_transmit)
  "transmit velocity, unit & direction converter"/2(velocity_motor0_out) -> serial communication/4(velocity_m0_transmit)
  "transmit velocity, unit & direction converter"/3(direction_motor1_out) -> serial communication/5(direction_m1_transmit)
  "transmit velocity, unit & direction converter"/4(velocity_motor1_out) -> serial communication/6(velocity_m1_transmit)
  "transmit velocity, unit & direction converter"/5(direction_motor2_out) -> serial communication/7(direction_m2_transmit)
  "transmit velocity, unit & direction converter"/6(velocity_motor2_out) -> serial communication/8(velocity_m2_transmit)
  v_x/1 -> "transmit velocity, unit & direction converter"/1(v_x_in)
  v_y/1 -> "transmit velocity, unit & direction converter"/2(v_y_in)
  v_theta/1 -> "transmit velocity, unit & direction converter"/3(v_theta_in)
  "receive direction, unit & velocity converter"/2(v_y_out) -> assemble robotino response/2(v_y_in), "v_Y_lokal "/1
  enable/1 -> serial communication/9(enable)
  serial communication/1(direction_motor0_receive) -> "receive direction, unit & velocity converter"/2(direction_motor0_in)
  serial communication/7(distance measuring sensors) -> distance converter/1(dms_in)
  serial communication/10(robotino raw data) -> Terminator/1
  serial communication/9(di03_bump) -> light barrier & slider/1(di03_bump_in)
  "receive direction, unit & velocity converter"/1(v_x_out) -> assemble robotino response/1(v_x_in), v_X_lokal/1
  "receive direction, unit & velocity converter"/3(v_theta_out) -> assemble robotino response/3(v_theta_in), "v_Psi_lokal "/1
  Grabber/1 -> Gain/1
  Gain/1 -> serial communication/1(dir)
  distance converter/1(dms_out) -> assemble robotino response/4(distance_measuring_sensors_in)
  light barrier & slider/2(slider) -> assemble robotino response/7(slider_in)
  light barrier & slider/1(light_barrier) -> assemble robotino response/6(light_barrier_in)
  serial communication/8(bumper) -> assemble robotino response/5(bumper_in)
  serial communication/2(velocity_motor0_receive) -> "receive direction, unit & velocity converter"/3(velocity_motor0_in)
  serial communication/3(direction_motor1_receive) -> "receive direction, unit & velocity converter"/4(direction_motor1_in)
  serial communication/4(velocity_motor1_receive) -> "receive direction, unit & velocity converter"/5(velocity_motor1_in)
  serial communication/5(direction_motor2_receive) -> "receive direction, unit & velocity converter"/6(direction_motor2_in)
  serial communication/6(velocity_motor2_receive) -> "receive direction, unit & velocity converter"/7(velocity_motor2_in)
  Grabber velocity/1 -> serial communication/2(vel)
  number of robot/1 -> "receive direction, unit & velocity converter"/1(number_of_robot)
  assemble robotino response/1(robotino_response) -> RobotinoDaten 1/1

== system Gesamtmodell_2015b/Regelung/Signal Builder ==
  Demux : Demux  Tag=STV Demux  Outputs=3
  FromWs : FromWorkspace  Tag=STV FromWs  VariableName=tuvar  SampleTime=0
      SigBuilderData=|
      | common.afterFinalStr = 'Extrapolate'
      | common.sampleTime = 0
      | dataSet.timeRange = [0 25]
      | dataSet.name = 'Group 1'
      | sbobj.Groups.Name = 'Group 1'
      | sbobj.Groups.Signals(1).Name = 'X Pos'
      | sbobj.Groups.Signals(1).XData = [0 5 7.5 10 12.5 25]
      | sbobj.Groups.Signals(1).YData = [5500 5500 6500 6500 5500 5500]
      | sbobj.Groups.Signals(2).Name = 'Y Pos'
      | sbobj.Groups.Signals(2).XData = [0 2.5 5 7.5 10 25]
      | sbobj.Groups.Signals(2).YData = [1000 1000 2000 2000 1000 1000]
      | sbobj.Groups.Signals(3).Name = 'Psi'
      | sbobj.Groups.Signals(3).XData = [0 2.5 5 7.5 10 20 25]
      | sbobj.Groups.Signals(3).YData = [0 0 3.14159265359 3.14159265359 0 0 0]
      | sbobj.Groups.TimeRange = [0 25]
  X Pos : Outport  Tag=STV Outport
  Y Pos : Outport  Tag=STV Outport  Port=2
  Psi : Outport  Tag=STV Outport  Port=3
  wires:
  FromWs/1 -> Demux/1
  Demux/1 -> X Pos/1
  Demux/2 -> Y Pos/1
  Demux/3 -> Psi/1

== system Gesamtmodell_2015b/Regelung/Signal Builder1 ==
  Demux : Demux  Tag=STV Demux  Outputs=3
  FromWs : FromWorkspace  Tag=STV FromWs  VariableName=tuvar  SampleTime=0
  X Pos : Outport  Tag=STV Outport
  Y Pos : Outport  Tag=STV Outport  Port=2
  Psi : Outport  Tag=STV Outport  Port=3
  wires:
  FromWs/1 -> Demux/1
  Demux/1 -> X Pos/1
  Demux/2 -> Y Pos/1
  Demux/3 -> Psi/1

== system Gesamtmodell_2015b/Regelung/Signal Builder2 ==
  Demux : Demux  Tag=STV Demux  Outputs=3
  FromWs : FromWorkspace  Tag=STV FromWs  VariableName=tuvar  SampleTime=0
      SigBuilderData=|
      | common.afterFinalStr = 'Extrapolate'
      | common.sampleTime = 0
      | dataSet.timeRange = [0 25]
      | dataSet.name = 'Group 1'
      | sbobj.Groups.Name = 'Group 1'
      | sbobj.Groups.Signals(1).Name = 'X Pos'
      | sbobj.Groups.Signals(1).XData = [0 2.5 5 10 12.5 25]
      | sbobj.Groups.Signals(1).YData = [5500 5500 5500 5500 5500 5500]
      | sbobj.Groups.Signals(2).Name = 'Y Pos'
      | sbobj.Groups.Signals(2).XData = [0 2.5 5 10 12.5 15 25]
      | sbobj.Groups.Signals(2).YData = [1000 1000 2000 2000 1000 1000 1000]
      | sbobj.Groups.Signals(3).Name = 'Psi'
      | sbobj.Groups.Signals(3).XData = [0 6 10 20 23.72 25]
      | sbobj.Groups.Signals(3).YData = [0 0 0 0 0 0]
      | sbobj.Groups.TimeRange = [0 25]
  X Pos : Outport  Tag=STV Outport
  Y Pos : Outport  Tag=STV Outport  Port=2
  Psi : Outport  Tag=STV Outport  Port=3
  wires:
  FromWs/1 -> Demux/1
  Demux/1 -> X Pos/1
  Demux/2 -> Y Pos/1
  Demux/3 -> Psi/1

== system Gesamtmodell_2015b/Regelung/Signal Builder3 ==
  Demux : Demux  Tag=STV Demux  Outputs=3
  FromWs : FromWorkspace  Tag=STV FromWs  VariableName=tuvar  SampleTime=0
      SigBuilderData=|
      | common.afterFinalStr = 'Extrapolate'
      | common.sampleTime = 0
      | dataSet.timeRange = [0 45]
      | dataSet.name = 'Group 1'
      | sbobj.Groups.Name = 'Group 1'
      | sbobj.Groups.Signals(1).Name = 'X Pos'
      | sbobj.Groups.Signals(1).XData = [0 5 10 15 20 24.95 30.05 35 40 45]
      | sbobj.Groups.Signals(1).YData = [1400 1400 1900 2400 2400 2400 2400 1900 1400 1400]
      | sbobj.Groups.Signals(2).Name = 'Y Pos'
      | sbobj.Groups.Signals(2).XData = [0 0.55 5 10 15 19.95 25 29.95 35 40 45]
      | sbobj.Groups.Signals(2).YData = [1000 1000 1500 1500 1500 1500 1250 1000 1000 1000 1000]
      | sbobj.Groups.Signals(3).Name = 'Psi'
      | sbobj.Groups.Signals(3).XData = [0 5 10 15 20 25 30 35.1 40 45]
      | sbobj.Groups.Signals(3).YData = [1.5708 1.5708 6.28318530718 3.14 0 0 -3.14159265359 3.14159265359 0 0]
      | sbobj.Groups.TimeRange = [0 45]
  X Pos : Outport  Tag=STV Outport
  Y Pos : Outport  Tag=STV Outport  Port=2
  Psi : Outport  Tag=STV Outport  Port=3
  wires:
  Demux/3 -> Psi/1
  Demux/2 -> Y Pos/1
  Demux/1 -> X Pos/1
  FromWs/1 -> Demux/1

== system Gesamtmodell_2015b/Regelung/Signal Builder4 ==
  Demux : Demux  Tag=STV Demux  Outputs=3
  FromWs : FromWorkspace  Tag=STV FromWs  VariableName=tuvar  SampleTime=0
      SigBuilderData=|
      | common.afterFinalStr = 'Extrapolate'
      | common.sampleTime = 0
      | dataSet.timeRange = [0 45]
      | dataSet.name = 'Group 1'
      | sbobj.Groups.Name = 'Group 1'
      | sbobj.Groups.Signals(1).Name = 'X Pos'
      | sbobj.Groups.Signals(1).XData = [0 5 10 15 20 24.95 30.05 35 40 45]
      | sbobj.Groups.Signals(1).YData = [3400 3400 3900 4400 4400 4400 4400 3900 3400 3400]
      | sbobj.Groups.Signals(2).Name = 'Y Pos'
      | sbobj.Groups.Signals(2).XData = [0 0.55 5 10 15 19.95 25 29.95 35 40 45]
      | sbobj.Groups.Signals(2).YData = [1000 1000 1500 1500 1500 1500 1250 1000 1000 1000 1000]
      | sbobj.Groups.Signals(3).Name = 'Psi'
      | sbobj.Groups.Signals(3).XData = [0 5 10 15 20 25 30 35.1 40 45]
      | sbobj.Groups.Signals(3).YData = [1.5708 1.5708 6.28318530718 3.14 0 0 -3.14159265359 3.14159265359 0 0]
      | sbobj.Groups.TimeRange = [0 45]
  X Pos : Outport  Tag=STV Outport
  Y Pos : Outport  Tag=STV Outport  Port=2
  Psi : Outport  Tag=STV Outport  Port=3
  wires:
  Demux/3 -> Psi/1
  Demux/2 -> Y Pos/1
  Demux/1 -> X Pos/1
  FromWs/1 -> Demux/1

== system Gesamtmodell_2015b/Regelung/Signal Builder5 ==
  Demux : Demux  Tag=STV Demux  Outputs=3
  FromWs : FromWorkspace  Tag=STV FromWs  VariableName=tuvar  SampleTime=0
      SigBuilderData=|
      | common.afterFinalStr = 'Extrapolate'
      | common.sampleTime = 0
      | dataSet.timeRange = [0 45]
      | dataSet.name = 'Group 1'
      | sbobj.Groups.Name = 'Group 1'
      | sbobj.Groups.Signals(1).Name = 'X Pos'
      | sbobj.Groups.Signals(1).XData = [0 5 10 15 20 24.95 30.05 35 40 45]
      | sbobj.Groups.Signals(1).YData = [5300 4850 4100 3200 2850 2250 1900 1650 1400 750]
      | sbobj.Groups.Signals(2).Name = 'Y Pos'
      | sbobj.Groups.Signals(2).XData = [0 0.55 5 10 15 19.95 25 29.95 35 40 45]
      | sbobj.Groups.Signals(2).YData = [3450 3450 3450 3450 3450 3450 3450 3450 3450 3450 3450]
      | sbobj.Groups.Signals(3).Name = 'Psi'
      | sbobj.Groups.Signals(3).XData = [0 5 10 15 20 25 30 35.1 40 45]
      | sbobj.Groups.Signals(3).YData = [1.57079632679 1.56 1.54 0 0 -1.57079632679 -1.5 -1.46 0 0]
      | sbobj.Groups.TimeRange = [0 45]
  X Pos : Outport  Tag=STV Outport
  Y Pos : Outport  Tag=STV Outport  Port=2
  Psi : Outport  Tag=STV Outport  Port=3
  wires:
  Demux/3 -> Psi/1
  Demux/2 -> Y Pos/1
  Demux/1 -> X Pos/1
  FromWs/1 -> Demux/1

== system Gesamtmodell_2015b/Regelung/Stellgrößen- beschränkung  ==
  note: in rad/sec
  note: in mm/sec
  note: in mm/sec
  vX : Inport
  vY : Inport  Port=2
  vPsi : Inport  Port=3
  "Beschraenkung " : MATLAB Function  TreatAsAtomicUnit=on
  MaxStellR : Constant  Value=5
  MaxStellT : Constant  Value=400
  vXlim : Outport
  vYlim : Outport  Port=2
  vPsiLim : Outport  Port=3
  wires:
  MaxStellT/1 -> "Beschraenkung "/1(MaxStellT)
  "Beschraenkung "/1(X) -> vXlim/1
  "Beschraenkung "/2(Y) -> vYlim/1
  "Beschraenkung "/3(Theta) -> vPsiLim/1
  MaxStellR/1 -> "Beschraenkung "/2(MaxStellR)
  vX/1 -> "Beschraenkung "/3(x)
  vY/1 -> "Beschraenkung "/4(y)
  vPsi/1 -> "Beschraenkung "/5(theta)

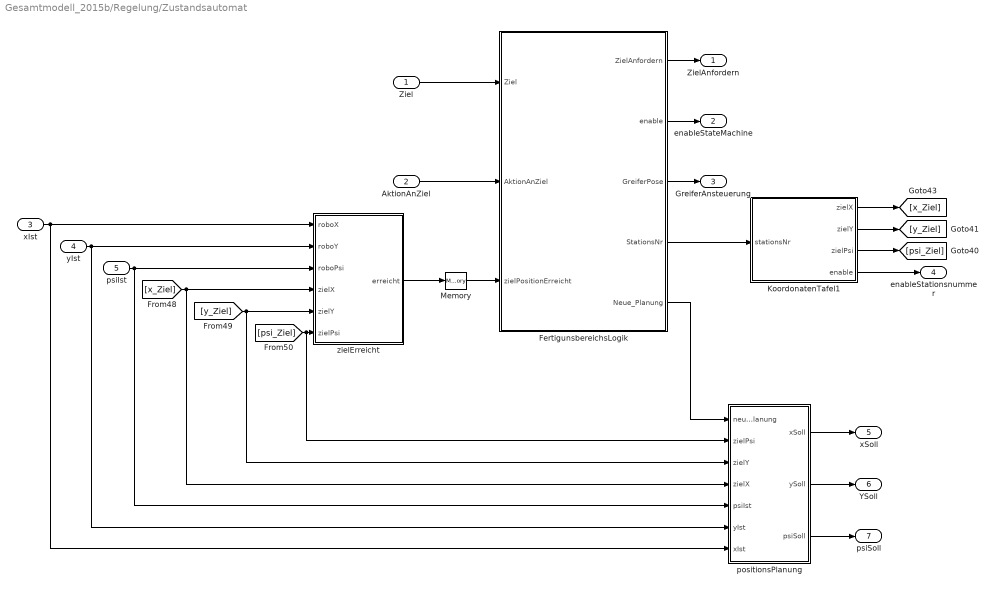
== system Gesamtmodell_2015b/Regelung/Zustandsautomat ==
  "Ziel " : Inport
  AktionAnZiel : Inport  Port=2
  xIst : Inport  Port=3
  yIst : Inport  Port=4
  psiIst : Inport  Port=5
  FertigunsbereichsLogik : Stateflow chart  TreatAsAtomicUnit=on
  KoordonatenTafel1 : MATLAB Function  TreatAsAtomicUnit=on
  Memory : Memory
  positionsPlanung : MATLAB Function  TreatAsAtomicUnit=on
  zielErreicht : MATLAB Function  TreatAsAtomicUnit=on
  ZielAnfordern : Outport
  enableStateMachine : Outport  Port=2
  GreiferAnsteuerung : Outport  Port=3
  enableStationsnummer : Outport  Port=4
  xSoll : Outport  Port=5
  YSoll : Outport  Port=6
  psiSoll : Outport  Port=7
  wires:
  [y_Ziel] -> positionsPlanung/3(zielY), zielErreicht/5(zielY)
  psiIst/1 -> positionsPlanung/5(psiIst), zielErreicht/3(roboPsi)
  KoordonatenTafel1/4(enable) -> enableStationsnummer/1
  AktionAnZiel/1 -> FertigunsbereichsLogik/2(AktionAnZiel)
  [psi_Ziel] -> positionsPlanung/2(zielPsi), zielErreicht/6(zielPsi)
  positionsPlanung/1(xSoll) -> xSoll/1
  positionsPlanung/2(ySoll) -> YSoll/1
  yIst/1 -> zielErreicht/2(roboY), positionsPlanung/6(yIst)
  FertigunsbereichsLogik/2(enable) -> enableStateMachine/1
  FertigunsbereichsLogik/4(StationsNr) -> KoordonatenTafel1/1(stationsNr)
  [x_Ziel] -> positionsPlanung/4(zielX), zielErreicht/4(zielX)
  positionsPlanung/3(psiSoll) -> psiSoll/1
  Memory/1 -> FertigunsbereichsLogik/3(zielPositionErreicht)
  "Ziel "/1 -> FertigunsbereichsLogik/1(Ziel)
  xIst/1 -> zielErreicht/1(roboX), positionsPlanung/7(xIst)
  zielErreicht/1(erreicht) -> Memory/1
  FertigunsbereichsLogik/5(Neue_Planung) -> positionsPlanung/1(neuePlanung)
  FertigunsbereichsLogik/1(ZielAnfordern) -> ZielAnfordern/1
  FertigunsbereichsLogik/3(GreiferPose) -> GreiferAnsteuerung/1
  KoordonatenTafel1/1(zielX) -> [x_Ziel]
  KoordonatenTafel1/2(zielY) -> [y_Ziel]
  KoordonatenTafel1/3(zielPsi) -> [psi_Ziel]

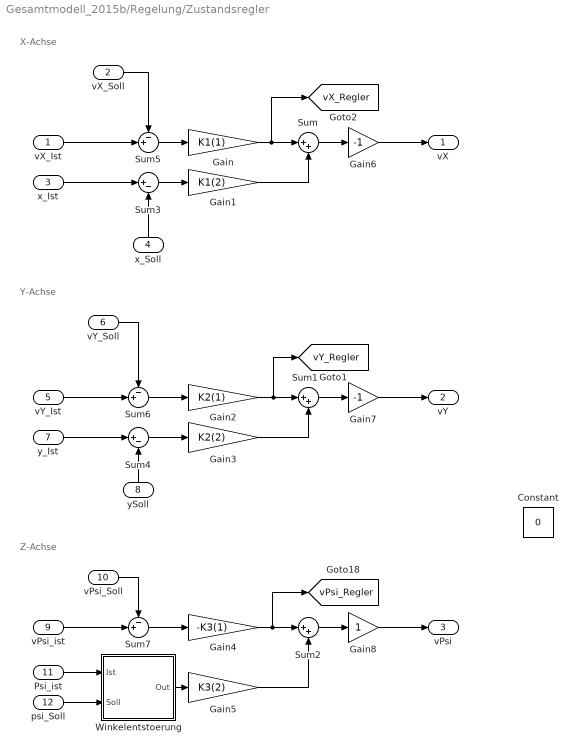
== system Gesamtmodell_2015b/Regelung/Zustandsregler ==
  note: Z-Achse
  note: Y-Achse
  note: X-Achse
  vX_Ist : Inport
  "vX_Soll " : Inport  Port=2
  x_Ist : Inport  Port=3
  x_Soll : Inport  Port=4
  vY_Ist : Inport  Port=5
  "vY_Soll " : Inport  Port=6
  y_Ist : Inport  Port=7
  ySoll : Inport  Port=8
  vPsi_ist : Inport  Port=9
  vPsi_Soll : Inport  Port=10
  Psi_ist : Inport  Port=11
  "psi_Soll " : Inport  Port=12
  Constant : Constant  Value=0
  Gain : Gain  Gain=K1(1)
  Gain1 : Gain  Gain=K1(2)
  Gain2 : Gain  Gain=K2(1)
  Gain3 : Gain  Gain=K2(2)
  Gain4 : Gain  Gain=-K3(1)
  Gain5 : Gain  Gain=K3(2)
  Gain6 : Gain  Gain=-1
  Gain7 : Gain  Gain=-1
  Gain8 : Gain
  Sum : Sum  Inputs=|++
  Sum1 : Sum  Inputs=|++
  Sum2 : Sum  Inputs=|++
  Sum3 : Sum  Inputs=|+-
  Sum4 : Sum  Inputs=|+-
  Sum5 : Sum  Inputs=-+|
  Sum6 : Sum  Inputs=-+|
  Sum7 : Sum  Inputs=-+|
  Winkelentstoerung : MATLAB Function  TreatAsAtomicUnit=on
  vX : Outport
  vY : Outport  Port=2
  "vPsi " : Outport  Port=3
  tag scope: vPsi_Regler=global, vX_Regler=global, vY_Regler=global
  wires:
  Gain/1 -> Sum/1, [vX_Regler]
  Gain1/1 -> Sum/2
  Gain2/1 -> [vY_Regler], Sum1/1
  Gain3/1 -> Sum1/2
  Gain4/1 -> Sum2/1, [vPsi_Regler]
  Gain5/1 -> Sum2/2
  Sum1/1 -> Gain7/1
  Sum/1 -> Gain6/1
  x_Ist/1 -> Sum3/1
  Sum3/1 -> Gain1/1
  y_Ist/1 -> Sum4/1
  Sum4/1 -> Gain3/1
  Gain6/1 -> vX/1
  Gain7/1 -> vY/1
  vPsi_ist/1 -> Sum7/2
  Sum2/1 -> Gain8/1
  Gain8/1 -> "vPsi "/1
  Psi_ist/1 -> Winkelentstoerung/1(Ist)
  vX_Ist/1 -> Sum5/2
  Sum5/1 -> Gain/1
  vY_Ist/1 -> Sum6/2
  Sum6/1 -> Gain2/1
  "vX_Soll "/1 -> Sum5/1
  "vY_Soll "/1 -> Sum6/1
  Sum7/1 -> Gain4/1
  vPsi_Soll/1 -> Sum7/1
  x_Soll/1 -> Sum3/2
  ySoll/1 -> Sum4/2
  "psi_Soll "/1 -> Winkelentstoerung/2(Soll)
  Winkelentstoerung/1(Out) -> Gain5/1

== system Gesamtmodell_2015b/Regelung/getRobotinoID ==
  note: Executing only once at start after 10ms
  Step : Step  Time=0.01  SampleTime=0
  getIDfromFlash : Subsystem
  Robotino.ID : Outport
  wires:
  Step/1 -> getIDfromFlash/Trigger
  getIDfromFlash/1(RobotinoID) -> Robotino.ID/1

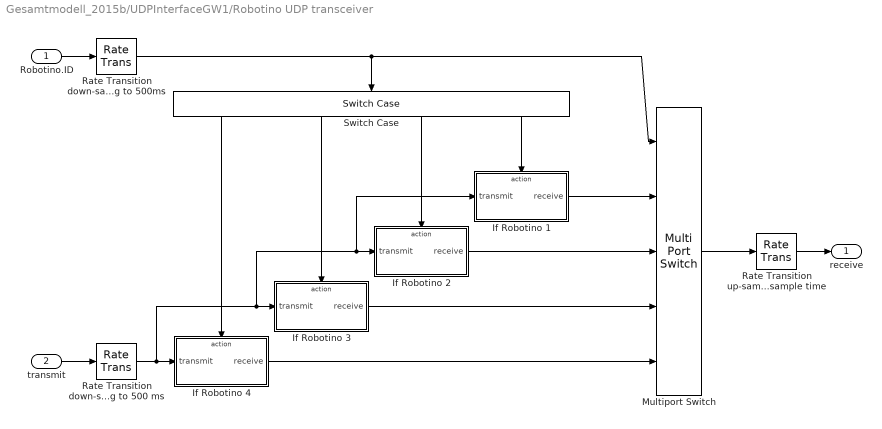
== system Gesamtmodell_2015b/UDPInterfaceGW1/Robotino UDP transceiver ==
  Robotino.ID : Inport
  transmit : Inport  Port=2
  If Robotino 1 : Subsystem  TreatAsAtomicUnit=on
  If Robotino 2 : Subsystem  TreatAsAtomicUnit=on
  If Robotino 3 : Subsystem  TreatAsAtomicUnit=on
  If Robotino 4 : Subsystem  TreatAsAtomicUnit=on
  Multiport Switch : MultiPortSwitch  Inputs=4
  Rate Transition down-sampling to 500 ms : RateTransition  OutPortSampleTime=0.5
  Rate Transition down-sampling to 500ms : RateTransition  OutPortSampleTime=0.5
  Rate Transition up-sampling to fundamental sample time : RateTransition
  Switch Case : SwitchCase  CaseConditions={4,3,2,1}  ShowDefaultCase=off
  receive : Outport
  wires:
  Switch Case/1 -> If Robotino 4/Action
  Switch Case/2 -> If Robotino 3/Action
  Switch Case/3 -> If Robotino 2/Action
  Switch Case/4 -> If Robotino 1/Action
  Multiport Switch/1 -> Rate Transition up-sampling to fundamental sample time/1
  If Robotino 1/1(receive) -> Multiport Switch/2
  If Robotino 3/1(receive) -> Multiport Switch/4
  If Robotino 2/1(receive) -> Multiport Switch/3
  If Robotino 4/1(receive) -> Multiport Switch/5
  transmit/1 -> Rate Transition down-sampling to 500 ms/1
  Rate Transition up-sampling to fundamental sample time/1 -> receive/1
  Rate Transition down-sampling to 500 ms/1 -> If Robotino 4/1(transmit), If Robotino 3/1(transmit), If Robotino 2/1(transmit), If Robotino 1/1(transmit)
  Robotino.ID/1 -> Rate Transition down-sampling to 500ms/1
  Rate Transition down-sampling to 500ms/1 -> Switch Case/1, Multiport Switch/1

== system Gesamtmodell_2015b/Regelung/Receiver/UDP interface ==
  number of robot : Inport
  Receive : xpcrtudplib/Legacy UDP/Receive   ipAddress=0.0.0.0  ipPort=25000  width=448  vblLen=off  sampletime=-1
  Terminator : Terminator
  Unpack : xpcobsoletelib/Utilities/Unpack   dimensions={[56]}  datatypes={'double'}  byteAlign=1
  stop signals : MATLAB Function  TreatAsAtomicUnit=on
  enable : Outport
  UDP data : Outport  Port=2
  wires:
  Unpack/1 -> stop signals/2(udp_in), UDP data/1
  Receive/1 -> Unpack/1
  Receive/2 -> Terminator/1
  stop signals/1(enable_out) -> enable/1
  number of robot/1 -> stop signals/1(rob_number)

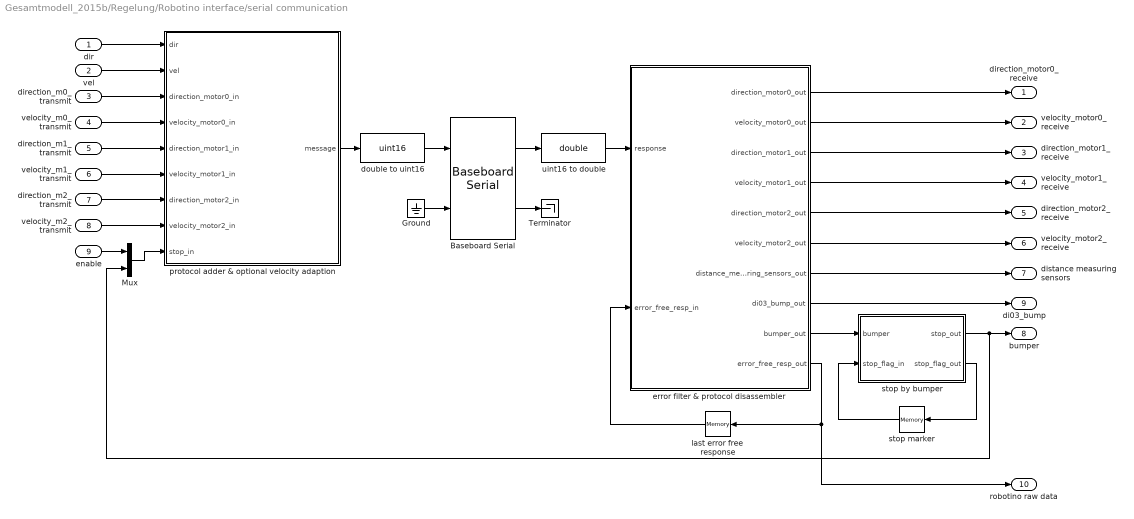
== system Gesamtmodell_2015b/Regelung/Robotino interface/serial communication ==
  dir : Inport
  vel : Inport  Port=2
  direction_m0_transmit : Inport  Port=3
  velocity_m0_transmit : Inport  Port=4
  direction_m1_transmit : Inport  Port=5
  velocity_m1_transmit : Inport  Port=6
  direction_m2_transmit : Inport  Port=7
  velocity_m2_transmit : Inport  Port=8
  enable : Inport  Port=9
  Baseboard Serial : xpcseriallib/Mainboard/Baseboard Serial  group=Transmit Setup  port=2  irqnum=4  saddr1=0x3f8  saddr2=0x3e8  config=Com1/none  baud1=115200  parity1=None  ndata1=8  nstop1=1  fifomode1=16 deep  rlevel1=almost full  automode1=off  xmtfifosize1=10240  xmtdatatype1=count+16 bit uint  rcvfifosize1=10240  rcvmaxread1=101  rcvminread1=1  rcvusedelim1=on  rcvdelim1=99  rcvdatatype1=count+16 bit uint  rcvsampletime1=-1  baud2=115200  parity2=None  ndata2=8  nstop2=1  fifomode2=16 deep  rlevel2=almost full  automode2=off  xmtfifosize2=10240  xmtdatatype2=count+16 bit uint  rcvfifosize2=10240  rcvmaxread2=101  rcvminread2=1  rcvusedelim2=on  rcvdelim2=99  rcvdatatype2=count+16 bit uint  rcvsampletime2=-1
      link override FIFO read 1: maxsize=101  minsize=1  usedelimiter=on  delimiter=99  outputtype=count+16 bit uint  sampletime=dt / 2
      link override FIFO read 2: maxsize=101  minsize=1  usedelimiter=on  delimiter=99  outputtype=count+16 bit uint  sampletime=dt / 2
      link override FIFO write 1: size=1024  inputtype=count+16 bit uint  sampletime=-1  id=XMT channel 1, IRQ 4
      link override FIFO write 2: size=1024  inputtype=8 bit uint null terminated  id=XMT channel 2, IRQ 4
      link override Setup1: baud=115200  width=8  nstop=1  parity=None  fmode=16 deep  rlevel=half full  ctsmode=off
      link override Setup2: baud=4800  width=8  nstop=1  parity=None  fmode=16 deep  rlevel=half full  ctsmode=off
  Ground : Ground
  Mux : Mux  Inputs=2
  Terminator : Terminator
  double to uint16 : DataTypeConversion  OutDataTypeStr=uint16  RndMeth=Nearest
  error filter & protocol disassembler : MATLAB Function  TreatAsAtomicUnit=on
  last error free response : Memory  X0=[zeros(1,102)]
  protocol adder & optional velocity adaption : MATLAB Function  TreatAsAtomicUnit=on
  stop by bumper : MATLAB Function  TreatAsAtomicUnit=on
  stop marker : Memory  X0=[zeros(1,3)]
  uint16 to double : DataTypeConversion  OutDataTypeStr=double  RndMeth=Nearest
  direction_motor0_receive : Outport
  velocity_motor0_receive : Outport  Port=2
  direction_motor1_receive : Outport  Port=3
  velocity_motor1_receive : Outport  Port=4
  direction_motor2_receive : Outport  Port=5
  velocity_motor2_receive : Outport  Port=6
  distance measuring sensors : Outport  Port=7
  bumper : Outport  Port=8
  di03_bump : Outport  Port=9
  robotino raw data : Outport  Port=10
  wires:
  Ground/1 -> Baseboard Serial/2
  Baseboard Serial/2 -> Terminator/1
  double to uint16/1 -> Baseboard Serial/1
  protocol adder & optional velocity adaption/1(message) -> double to uint16/1
  stop marker/1 -> stop by bumper/2(stop_flag_in)
  stop by bumper/2(stop_flag_out) -> stop marker/1
  last error free response/1 -> error filter & protocol disassembler/2(error_free_resp_in)
  error filter & protocol disassembler/10(error_free_resp_out) -> last error free response/1, robotino raw data/1
  error filter & protocol disassembler/1(direction_motor0_out) -> direction_motor0_receive/1
  error filter & protocol disassembler/2(velocity_motor0_out) -> velocity_motor0_receive/1
  error filter & protocol disassembler/3(direction_motor1_out) -> direction_motor1_receive/1
  error filter & protocol disassembler/4(velocity_motor1_out) -> velocity_motor1_receive/1
  direction_m0_transmit/1 -> protocol adder & optional velocity adaption/3(direction_motor0_in)
  error filter & protocol disassembler/5(direction_motor2_out) -> direction_motor2_receive/1
  velocity_m0_transmit/1 -> protocol adder & optional velocity adaption/4(velocity_motor0_in)
  error filter & protocol disassembler/6(velocity_motor2_out) -> velocity_motor2_receive/1
  direction_m1_transmit/1 -> protocol adder & optional velocity adaption/5(direction_motor1_in)
  velocity_m1_transmit/1 -> protocol adder & optional velocity adaption/6(velocity_motor1_in)
  direction_m2_transmit/1 -> protocol adder & optional velocity adaption/7(direction_motor2_in)
  velocity_m2_transmit/1 -> protocol adder & optional velocity adaption/8(velocity_motor2_in)
  error filter & protocol disassembler/9(bumper_out) -> stop by bumper/1(bumper)
  stop by bumper/1(stop_out) -> bumper/1, Mux/2
  error filter & protocol disassembler/7(distance_measuring_sensors_out) -> distance measuring sensors/1
  Baseboard Serial/1 -> uint16 to double/1
  uint16 to double/1 -> error filter & protocol disassembler/1(response)
  enable/1 -> Mux/1
  dir/1 -> protocol adder & optional velocity adaption/1(dir)
  vel/1 -> protocol adder & optional velocity adaption/2(vel)
  Mux/1 -> protocol adder & optional velocity adaption/9(stop_in)
  error filter & protocol disassembler/8(di03_bump_out) -> di03_bump/1

== system Gesamtmodell_2015b/Regelung/getRobotinoID/getIDfromFlash ==
  Trigger : TriggerPort
  From File : slrtlib/Target Management/From File   filename='robotino.id'  dataSize=8  bufSize=2000  readSize=512  EOFOption=Seek to beginning  sampTime=-1  show2ports=off
  Unpack : xpcobsoletelib/Utilities/Unpack   dimensions={[1]}  datatypes={'double'}  byteAlign=1
  RobotinoID : Outport
  wires:
  From File/1 -> Unpack/1
  Unpack/1 -> RobotinoID/1

== system Gesamtmodell_2015b/UDPInterfaceGW1/Robotino UDP transceiver/If Robotino 1 ==
  transmit : Inport
  Action Port : ActionPort  ActionType=case
  Receive from all : xpcrtudplib/Legacy UDP/Receive   ipAddress=0.0.0.0  ipPort=25011  width=8  vblLen=off  sampletime=-1
  Send to all : xpcrtudplib/Legacy UDP/Send   ipAddress=255.255.255.255  ipPort=25010  localPort=-1  vblLen=off  sampletime=-1
  Terminator : Terminator
  receive : Outport
  wires:
  Receive from all/1 -> receive/1
  Receive from all/2 -> Terminator/1
  transmit/1 -> Send to all/1

== system Gesamtmodell_2015b/UDPInterfaceGW1/Robotino UDP transceiver/If Robotino 2 ==
  transmit : Inport
  Action Port : ActionPort  ActionType=case
  Receive from all : xpcrtudplib/Legacy UDP/Receive   ipAddress=0.0.0.0  ipPort=25012  width=8  vblLen=off  sampletime=-1
  Send to all : xpcrtudplib/Legacy UDP/Send   ipAddress=255.255.255.255  ipPort=25020  localPort=-1  vblLen=off  sampletime=-1
  Terminator : Terminator
  receive : Outport
  wires:
  Receive from all/1 -> receive/1
  Receive from all/2 -> Terminator/1
  transmit/1 -> Send to all/1

== system Gesamtmodell_2015b/UDPInterfaceGW1/Robotino UDP transceiver/If Robotino 3 ==
  transmit : Inport
  Action Port : ActionPort  ActionType=case
  Receive from all : xpcrtudplib/Legacy UDP/Receive   ipAddress=0.0.0.0  ipPort=25013  width=8  vblLen=off  sampletime=-1
  Send to all : xpcrtudplib/Legacy UDP/Send   ipAddress=255.255.255.255  ipPort=25030  localPort=-1  vblLen=off  sampletime=-1
  Terminator : Terminator
  receive : Outport
  wires:
  Receive from all/1 -> receive/1
  Receive from all/2 -> Terminator/1
  transmit/1 -> Send to all/1

== system Gesamtmodell_2015b/UDPInterfaceGW1/Robotino UDP transceiver/If Robotino 4 ==
  transmit : Inport
  Action Port : ActionPort  ActionType=case
  Receive from all : xpcrtudplib/Legacy UDP/Receive   ipAddress=0.0.0.0  ipPort=25014  width=8  vblLen=off  sampletime=-1
  Send to all : xpcrtudplib/Legacy UDP/Send   ipAddress=255.255.255.255  ipPort=25040  localPort=-1  vblLen=off  sampletime=-1
  Terminator : Terminator
  receive : Outport
  wires:
  Receive from all/1 -> receive/1
  Receive from all/2 -> Terminator/1
  transmit/1 -> Send to all/1
